simulink model "tmp"  (R2022b)
settings: Solver=VariableStepAuto  StartTime=0.0  StopTime=10.0  RelTol=1e-3
settings Model: Creator=chris  LastModifiedBy=chris

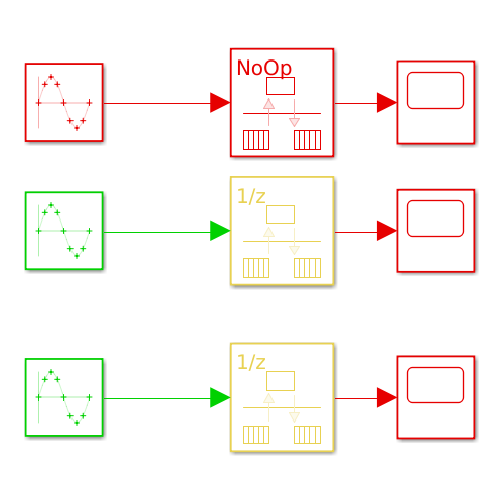
[thumbnail: Simulink's stored preview of the top-level diagram]
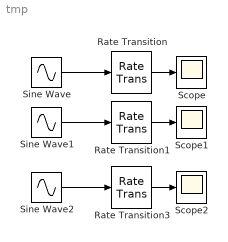
== system tmp ==
  Rate Transition : RateTransition
  Rate Transition1 : RateTransition  InitialCondition=10
  Rate Transition3 : RateTransition
  Scope : Scope
  Scope1 : Scope
  Scope2 : Scope
  Sine Wave : Sin  SineType=Sample based  SampleTime=0.01
  Sine Wave1 : Sin  SineType=Sample based  SampleTime=0.1
  Sine Wave2 : Sin  SineType=Sample based  SampleTime=0.1
  wires:
  Sine Wave/1 -> Rate Transition/1
  Sine Wave1/1 -> Rate Transition1/1
  Rate Transition/1 -> Scope/1
  Rate Transition1/1 -> Scope1/1
  Sine Wave2/1 -> Rate Transition3/1
  Rate Transition3/1 -> Scope2/1
